simulink model "MotorAsincronoMotorCC1"  (Simulink 8.5)
settings: Solver=ode23t  StartTime=0.0  StopTime=3  RelTol=1e-3
undefined symbols (not defined in the file): powergui
libraries: powerlib x28, powerlib_extras x3
settings Model: Creator=RS  LastModifiedBy=Diego Cisternas
settings OptimizationCC: ExpressionDepthLimit=128  InitFltsAndDblsToZero=on
settings DebuggingCC: SaveWithParameterizedLinksMsg=none  SignalResolutionControl=TryResolveAllWithWarning  SolverPrmCheckMsg=warning  FcnCallInpInsideContextMsg=UseLocalSettings  StateNameClashWarn=none  StrictBusMsg=Warning
settings GRTTargetCC: TargetFcnLib=ansi_tfl_tmw.mat

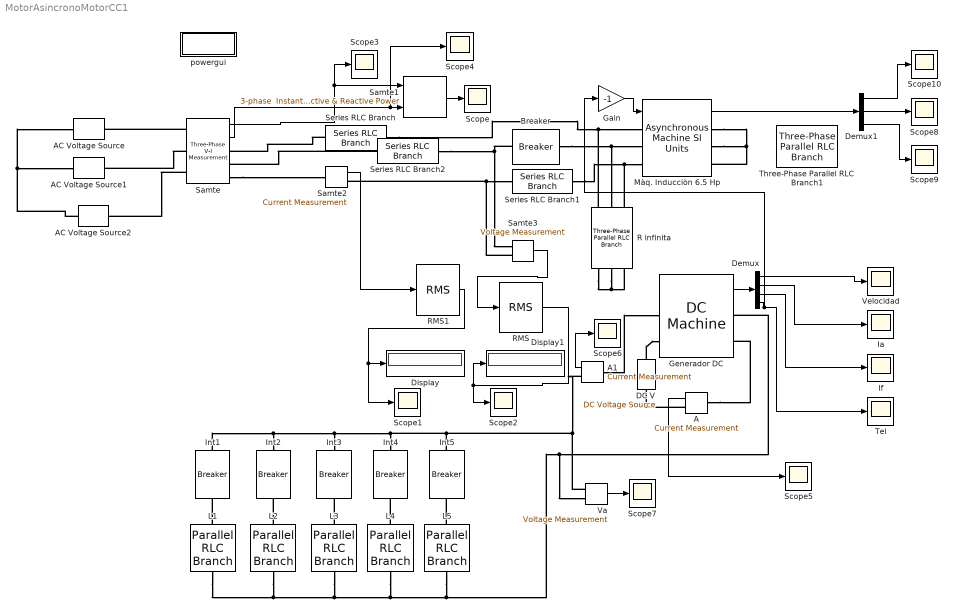
== system MotorAsincronoMotorCC1 ==
  A : powerlib/Measurements/Current Measurement  PhasorSimulation=off  OutputType=Complex  PSBequivalent=0
  A1 : powerlib/Measurements/Current Measurement  PhasorSimulation=off  OutputType=Complex  PSBequivalent=0
  AC Voltage Source : powerlib/Electrical Sources/AC Voltage Source  Amplitude=220.7*sqrt(2)  Phase=0  Frequency=50  SampleTime=0  Measurements=None
  AC Voltage Source1 : powerlib/Electrical Sources/AC Voltage Source  Amplitude=218.7*sqrt(2)  Phase=-119.5  Frequency=50  SampleTime=0  Measurements=None
  AC Voltage Source2 : powerlib/Electrical Sources/AC Voltage Source  Amplitude=220.7*sqrt(2)  Phase=121.3  Frequency=50  SampleTime=0  Measurements=None
  Breaker : powerlib/Elements/Breaker  InitialState=1  SwitchingTimes=0.7  External=off  BreakerResistance=0.01  SnubberResistance=1e6  SnubberCapacitance=inf  Measurements=None  MoreParameters=off  NoBreakLoop=off
  DC V : powerlib/Electrical Sources/DC Voltage Source  Amplitude=190  Measurements=None
  Demux : Demux
  Demux1 : Demux  Outputs=3
  Display : Display
  Display1 : Display
  Gain : Gain  Gain=-1
  Generador DC : powerlib/Machines/DC Machine  PresetModel=No  MechanicalLoad=Speed w  FieldType=Wound  ShowDetailedParameters=on  MeasurementBus=off  RLa="[ 0.5  0.01]"  RLf="[ 240  120]"  Laf=1.8  MachineConstant=Torque constant (N.m/A)  Ke=1.8  Kt=1.8  J=0.05  Bm=0.02  Tf=0  w0=0  Ifinit=1  TsPowergui=0  TsBlock=-1
  Ia : Scope
      settings: TimeRange=3  SaveName=ScopeData4  MaxDataPoints=10000000  SampleInput=on  SampleTime=10e-6
  If : Scope
      settings: SaveName=ScopeData5  MaxDataPoints=10000000  SampleInput=on  SampleTime=10e-6
  Int1 : powerlib/Elements/Breaker  InitialState=0  SwitchingTimes=0  External=off  BreakerResistance=0.01  SnubberResistance=1e6  SnubberCapacitance=inf  Measurements=None  MoreParameters=off  NoBreakLoop=off
  Int{2..5} (4 alike) : powerlib/Elements/Breaker  InitialState=0  SwitchingTimes=5  External=off  BreakerResistance=0.01  SnubberResistance=1e6  SnubberCapacitance=inf  Measurements=None  MoreParameters=off  NoBreakLoop=off
  L1 : powerlib/Elements/Parallel RLC Branch  LConnTagsString=a  RConnTagsString=__new0  BranchType=R  Resistance=20  Inductance=1e-3  SetiL0=off  InitialCurrent=0  Capacitance=1e-6  Setx0=off  InitialVoltage=0  Measurements=None
  L{2..5} (4 alike) : powerlib/Elements/Parallel RLC Branch  LConnTagsString=a  RConnTagsString=__new0  BranchType=R  Resistance=40  Inductance=1e-3  SetiL0=off  InitialCurrent=0  Capacitance=1e-6  Setx0=off  InitialVoltage=0  Measurements=None
  Màq. Inducciòn 6.5 Hp : powerlib/Machines/Asynchronous Machine SI Units  RotorType=Wound  PresetModel=No  MechanicalLoad=Torque Tm  ShowDetailedParameters=on  ReferenceFrame=Stationary  Units=SI  MeasurementBus=off  NominalParameters="[6.5*746    380   50]"  Stator="[0.03   0.00006]"  Rotor="[1.094  0.00496]"  Cage1=[0.4155 0.002066]  Cage2=[0.4168 0.0003495]  Lm=0.105  Mechanical="[0.041    0.001   2]"  PolePairs=2  InitialConditions="[ 1,0   0,0,0   0,0,0 ]"  SimulateSaturation=on  Saturation=[ 0.5 3,6,9,12,15,18,30,50;20,190,380,400,420,440,450,451,452]  LoadFlowParameters=0  TsPowergui=0  TsBlock=-1  IterativeModel=Trapezoidal non iterative  Pmec=1.492e+006
  R infinita : powerlib/Elements/Three-Phase Parallel RLC Branch  LConnTagsString=A|B|C  RConnTagsString=A|B|C  BranchType=R  Resistance=1000000  Inductance=1e-3  Capacitance=1e-6  Measurements=None
  RMS : powerlib_extras/Measurements/RMS  f1=50
  RMS1 : powerlib_extras/Measurements/RMS  f1=50
  Samte : powerlib/Measurements/Three-Phase V-I Measurement  VoltageMeasurement=phase-to-phase  SetLabelV=off  LabelV=Vabc  Vpu=off  VpuLL=off  CurrentMeasurement=yes  SetLabelI=off  LabelI=Iabc  Ipu=off  Pbase=100e6  Vbase=500e3  OutputType=Complex  PhasorSimulation=off  PSBequivalent=0
  Samte1 : powerlib_extras/Measurements/3-phase  Instantaneous  Active & Reactive Power
  Samte2 : powerlib/Measurements/Current Measurement  PhasorSimulation=off  OutputType=Complex  PSBequivalent=0
  Samte3 : powerlib/Measurements/Voltage Measurement  PhasorSimulation=off  OutputType=Complex  PSBequivalent=0
  Scope{,1..10} (11 alike) : Scope
      Scope settings: MaxDataPoints=10000000  SampleInput=on  SampleTime=10e-6
      Scope1 settings: MaxDataPoints=10000000  SampleInput=on  SampleTime=10e-6
      Scope10 settings: SaveName=ScopeData14  MaxDataPoints=10000000  SampleInput=on  SampleTime=10e-6
      Scope2 settings: YMin=378.99  YMax=378.99  SaveName=ScopeData2  MaxDataPoints=10000000  SampleInput=on  SampleTime=10e-6
      Scope3 settings: SaveName=ScopeData10  MaxDataPoints=10000000  SampleInput=on  SampleTime=10e-6
      Scope4 settings: TimeRange=3  SaveName=ScopeData11  MaxDataPoints=10000000  SampleInput=on  SampleTime=10e-6
      Scope5 settings: YMin=-0.791667  YMax=-0.791667  SaveName=ScopeData12  MaxDataPoints=10000000  SampleInput=on  SampleTime=10e-6
      Scope6 settings: YMin=10.588  YMax=10.598  SaveName=ScopeData13  MaxDataPoints=10000000  SampleInput=on  SampleTime=10e-6
      Scope7 settings: YMin=168.4  YMax=169.9  SaveName=ScopeData7  MaxDataPoints=10000000  SampleInput=on  SampleTime=10e-6
      Scope8 settings: SaveName=ScopeData8  MaxDataPoints=10000000  SampleInput=on  SampleTime=10e-6
      Scope9 settings: SaveName=ScopeData9  MaxDataPoints=10000000  SampleInput=on  SampleTime=10e-6
  Series RLC Branch : powerlib/Elements/Series RLC Branch  LConnTagsString=__new0  RConnTagsString=__new0  BranchType=RL  Resistance=0.6  Inductance=0.0049  SetiL0=off  InitialCurrent=0  Capacitance=1e-6  Setx0=off  InitialVoltage=0  Measurements=None
  Series RLC Branch1 : powerlib/Elements/Series RLC Branch  LConnTagsString=__new0  RConnTagsString=__new0  BranchType=RL  Resistance=0.6  Inductance=0.0049  SetiL0=off  InitialCurrent=0  Capacitance=1e-6  Setx0=off  InitialVoltage=0  Measurements=None
  Series RLC Branch2 : powerlib/Elements/Series RLC Branch  LConnTagsString=__new0  RConnTagsString=__new0  BranchType=RL  Resistance=0.6  Inductance=0.0049  SetiL0=off  InitialCurrent=0  Capacitance=1e-6  Setx0=off  InitialVoltage=0  Measurements=None
  Tel : Scope
      settings: SaveName=ScopeData6  MaxDataPoints=10000000  SampleInput=on  SampleTime=10e-6
  Three-Phase Parallel RLC Branch1 : powerlib/Elements/Three-Phase Parallel RLC Branch  LConnTagsString=A|B|C  RConnTagsString=A|B|C  BranchType=R  Resistance=4.2  Inductance=1e-3  Capacitance=1e-6  Measurements=None
  Va : powerlib/Measurements/Voltage Measurement  PhasorSimulation=off  OutputType=Complex  PSBequivalent=0
  Velocidad : Scope
      settings: SaveName=ScopeData3  MaxDataPoints=10000000  SampleInput=on  SampleTime=10e-6
  powergui : Subsystem  AncestorBlock=powerlib/powergui  InitFcn=powergui( 'InitFcn_Callback' , gcb , 0 , [ ] );  mask(PSB option menu block){SimulationMode=Continuous, SampleTime=50e-6, echomessages=off, RestoreLinks=warning, x0status=blocks, Frange=[0:2:500], Ylog=off, Xlog=on, ShowGrid=off, save=off, variable=ZData, structure=, ZoomFFT=on, StartTime=0.0, cycles=1, DisplayStyle=1, fundamental=60, FreqAxis=off, MaxFrequency=1000, frequencyindice=50, frequencyindicesteady=1, RmsSteady=1, display=off, Ts=0, frequency=60, methode=off, HookPort=off, Interpol=off}
      mask prompts: SimulationMode "Simulation mode"; SampleTime "Sample time Ts (when simulation mode is Discrete) (s)"; echomessages "Echo  Messages"; RestoreLinks "Restore disabled links"; x0status "Initial electrical states status"; Frange "Impedance tool: Frequency Range"; Ylog "Impedance tool: Log impedance"; Xlog "Impedance tool: log Frequency"; ShowGrid "Impedance tool: grid"; save "Impedance tool: Save Data To Workspace"; variable "Impedance tool: Variable Name"; structure "Structure Name (PSBFFTSCOPE)"; ZoomFFT "ZoomFFT (PSBFFTSCOPE)"; StartTime "Start Time (PSBFFTSCOPE)"; cycles "Cycles (PSBFFTSCOPE)"; DisplayStyle "Display style (PSBFFTSCOPE)"; fundamental "Fundamental (PSBFFTSCOPE)"; FreqAxis "Frequency Axis (PSBFFTSCOPE)"; MaxFrequency "Max Frequency (PSBFFTSCOPE)"; frequencyindice "Load flow frequency (Hz)"; frequencyindicesteady "Frequency indice (STEADYSTATE)"; RmsSteady "RMS display (STEADYSTATE)"; display "Display Results"; Ts "OBSOLETE 1"; frequency "Phasor frequency (Hz)"; methode "Phasor simulation"; HookPort "Hook port"; Interpol "Interpolate"
      mask init:
      | powerlibroot = which('powersysdomain');
      | PSBroot = powerlibroot(1:end-16);
      | %
      | switch SimulationMode
      | 	case 1
      | 		message=sprintf('Continuous');
      | 	case 2
      |         SampleTimeeval=evalin('base',SampleTime,'NaN');
      |         if isnan(SampleTimeeval)
      |             message=sprintf('Warning !!,\nUndefined sample time');
      |         else
      |             message=sprintf('Discrete,\nTs = %.4g s.',SampleTimeeval);
      |         end
      | 	case 3
      | 		message=sprintf('Phasors');
      | end
      | if strcmp(bdroot,'powerlib')
      |   message='powergui';
      | end
      | power_initmask();
      settings: CopyFcn=powergui( 'Copy_Callback' , gcb , 0 , [ ] );  ModelCloseFcn=powergui( 'CloseButton_Callback' , gcb , [ ] , [ ] );  PreSaveFcn=powergui( 'CloseButton_Callback' , gcb , [ ] , [ ] );  NameChangeFcn=powergui( 'NameChangeFcn_Callback' , gcb , 0 , [ ] );
      settings: DeleteFcn=|
      | powergui( 'Copy_Callback' , gcb , 1 , [ ] );
      | powergui( 'CloseButton_Callback' , gcb , [ ] , [ ] );
      settings: OpenFcn=|
      | if (power_openblockproxy ('secondary'))
      | powergui(gcb,'PM')
      | end;
      mask Help: web(psbhelp)
      mask TypeOptions SimulationMode: Continuous | Discrete | Phasor
      mask TypeOptions RestoreLinks: yes | warning | no
      mask TypeOptions x0status: blocks | steady | zero
      mask Callback HookPort: powergui('HookPort',[],[],gcb);
      mask Display: disp(message)
  wires:
  Samte/1 -> Samte1/1, Scope3/1
  Samte/2 -> Samte1/2, Scope4/1
  Samte3/1 -> RMS/1
  RMS/1 -> Display1/1, Scope2/1
  Samte1/1 -> Scope/1
  Màq. Inducciòn 6.5 Hp/1 -> Demux1/1
  Generador DC/1 -> Demux/1
  Gain/1 -> Màq. Inducciòn 6.5 Hp/1
  Demux/4 -> Tel/1, Gain/1
  Demux/1 -> Velocidad/1
  Demux/2 -> Ia/1
  Demux/3 -> If/1
  Va/1 -> Scope7/1
  RMS1/1 -> Display/1, Scope1/1
  A/1 -> Scope5/1
  A1/1 -> Scope6/1
  Demux1/1 -> Scope10/1
  Samte2/1 -> RMS1/1
  Demux1/2 -> Scope8/1
  Demux1/3 -> Scope9/1
  connections:
  Breaker/LConn1 -- Series RLC Branch2/RConn1 -- Samte3/LConn1
  R infinita/LConn1 -- Series RLC Branch/RConn1 -- Màq. Inducciòn 6.5 Hp/LConn1
  Samte/LConn3 -- AC Voltage Source2/RConn1
  Samte/RConn3 -- Samte2/LConn1
  R infinita/LConn3 -- Màq. Inducciòn 6.5 Hp/LConn3 -- Series RLC Branch1/RConn1
  DC V/RConn1 -- Generador DC/LConn2
  L1/LConn1 -- Int1/RConn1
  L2/LConn1 -- Int2/RConn1
  L3/LConn1 -- Int3/RConn1
  L4/LConn1 -- Int4/RConn1
  L5/LConn1 -- Int5/RConn1
  L1/RConn1 -- L2/RConn1 -- L3/RConn1 -- L4/RConn1 -- L5/RConn1 -- Generador DC/RConn1 -- Va/LConn2
  Va/LConn1 -- A1/RConn1 -- Int1/LConn1 -- Int2/LConn1 -- Int3/LConn1 -- Int4/LConn1 -- Int5/LConn1
  R infinita/RConn1 -- R infinita/RConn3 -- R infinita/RConn2
  A/RConn1 -- DC V/LConn1
  A/LConn1 -- Generador DC/RConn2
  AC Voltage Source2/LConn1 -- AC Voltage Source/LConn1 -- AC Voltage Source1/LConn1
  Samte/LConn1 -- AC Voltage Source/RConn1
  Samte/LConn2 -- AC Voltage Source1/RConn1
  A1/LConn1 -- Generador DC/LConn1
  Breaker/RConn1 -- Màq. Inducciòn 6.5 Hp/LConn2 -- R infinita/LConn2
  Màq. Inducciòn 6.5 Hp/RConn1 -- Màq. Inducciòn 6.5 Hp/RConn3 -- Màq. Inducciòn 6.5 Hp/RConn2
  Series RLC Branch/LConn1 -- Samte/RConn1
  Samte3/LConn2 -- Series RLC Branch1/LConn1 -- Samte2/RConn1
  Series RLC Branch2/LConn1 -- Samte/RConn2

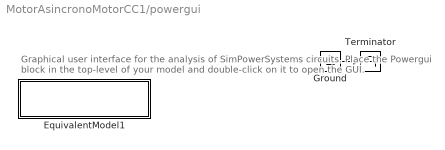
== system MotorAsincronoMotorCC1/powergui ==
  note: Graphical user interface for the analysis of  SimPowerSystems circuits.
      | Place the Powergui block in the top-level of your model and double-click
      | on it to open the GUI.
  EquivalentModel1 : Subsystem
      mask init:
      | SPS = get_param(gcbh,'UserData');
      | if isempty(SPS)
      |     A=0;
      |     B=0;
      |     C=0;
      |     D=0;
      |     x0=0;
      |     SwitchResistance=1;
      |     SwitchType=1;
      |     SwitchGateInitialValue=1;
      |     OutputsToResetToZero=1;
      | else
      | 	A=SPS.A;
      |     B=SPS.B;
      |     C=SPS.C;
      |     D=SPS.D;
      |     x0=SPS.x0;
      |     SwitchResistance=SPS.SwitchResistance;
      |     SwitchType=SPS.SwitchType;
      |     SwitchGateInitialValue=SPS.SwitchGateInitialValue;
      |     OutputsToResetToZero=SPS.YSwitchCurrent;
      | end
      mask Display:
      | color('blue')
      | disp('EQUIVALENT CIRCUIT')
  Ground : Ground
  Terminator : Terminator
  wires:
  Ground/1 -> Terminator/1

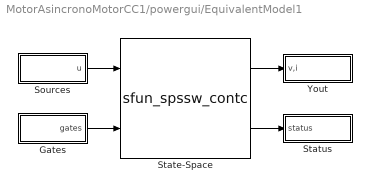
== system MotorAsincronoMotorCC1/powergui/EquivalentModel1 ==
  Gates : Subsystem
  Sources : Subsystem
  State-Space : S-Function  FunctionName=sfun_spssw_contc  Parameters=A, B, C, D, x0, SwitchResistance ,SwitchType, SwitchGateInitialValue, OutputsToResetToZero
  Status : Subsystem
  Yout : Subsystem
  wires:
  Gates/1(gates) -> State-Space/2
  Sources/1(u) -> State-Space/1
  State-Space/2 -> Status/1(status)
  State-Space/1 -> Yout/1(v,i)

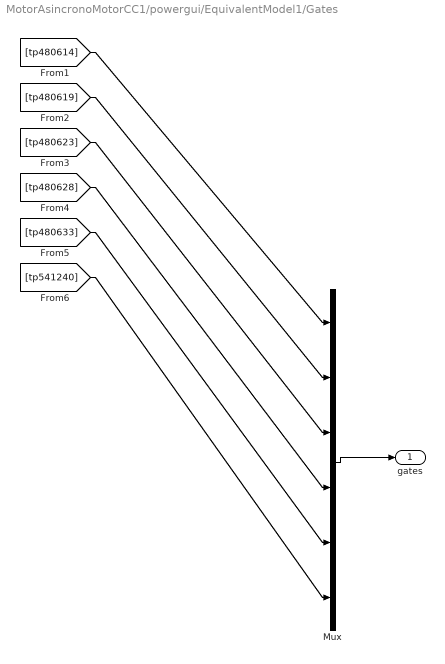
== system MotorAsincronoMotorCC1/powergui/EquivalentModel1/Gates ==
  Mux : Mux  Inputs=[1 1 1 1 1 1]
  gates : Outport
  wires:
  Mux/1 -> gates/1
  [tp480614] -> Mux/1
  [tp480619] -> Mux/2
  [tp480623] -> Mux/3
  [tp480628] -> Mux/4
  [tp480633] -> Mux/5
  [tp541240] -> Mux/6

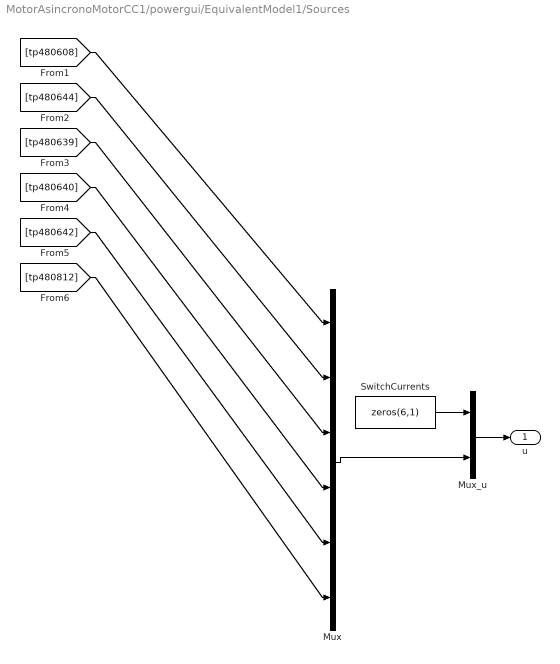
== system MotorAsincronoMotorCC1/powergui/EquivalentModel1/Sources ==
  Mux : Mux  Inputs=[4 1 1 1 1 1]
  Mux_u : Mux  Inputs=[6 9]
  SwitchCurrents : Constant  Value=zeros(6,1)
  u : Outport
  wires:
  Mux/1 -> Mux_u/2
  SwitchCurrents/1 -> Mux_u/1
  Mux_u/1 -> u/1
  [tp480608] -> Mux/1
  [tp480644] -> Mux/2
  [tp480639] -> Mux/3
  [tp480640] -> Mux/4
  [tp480642] -> Mux/5
  [tp480812] -> Mux/6

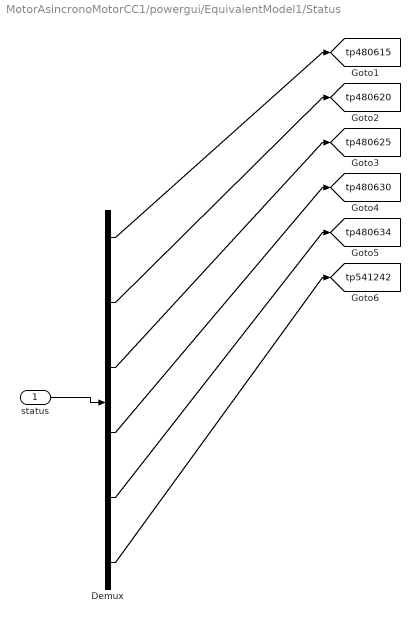
== system MotorAsincronoMotorCC1/powergui/EquivalentModel1/Status ==
  status : Inport
  Demux : Demux  Outputs=[1 1 1 1 1 1]
  tag scope: tp480615=global, tp480620=global, tp480625=global, tp480630=global, tp480634=global, tp541242=global
  wires:
  status/1 -> Demux/1
  Demux/1 -> [tp480615]
  Demux/2 -> [tp480620]
  Demux/3 -> [tp480625]
  Demux/4 -> [tp480630]
  Demux/5 -> [tp480634]
  Demux/6 -> [tp541242]

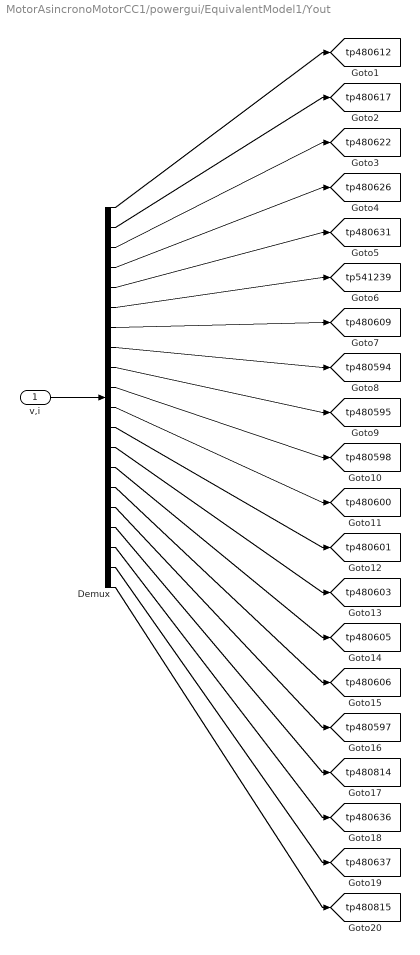
== system MotorAsincronoMotorCC1/powergui/EquivalentModel1/Yout ==
  v,i : Inport
  Demux : Demux  Outputs=[1 1 1 1 1 1 4 1 1 1 1 1 1 1 1 1 1 1 1 1]
  tag scope: tp480594=global, tp480595=global, tp480597=global, tp480598=global, tp480600=global, tp480601=global, tp480603=global, tp480605=global, tp480606=global, tp480609=global, tp480612=global, tp480617=global, tp480622=global, tp480626=global, tp480631=global, tp480636=global, tp480637=global, tp480814=global, tp480815=global, tp541239=global
  wires:
  v,i/1 -> Demux/1
  Demux/1 -> [tp480612]
  Demux/2 -> [tp480617]
  Demux/3 -> [tp480622]
  Demux/4 -> [tp480626]
  Demux/5 -> [tp480631]
  Demux/6 -> [tp541239]
  Demux/7 -> [tp480609]
  Demux/8 -> [tp480594]
  Demux/9 -> [tp480595]
  Demux/10 -> [tp480598]
  Demux/11 -> [tp480600]
  Demux/12 -> [tp480601]
  Demux/13 -> [tp480603]
  Demux/14 -> [tp480605]
  Demux/15 -> [tp480606]
  Demux/16 -> [tp480597]
  Demux/17 -> [tp480814]
  Demux/18 -> [tp480636]
  Demux/19 -> [tp480637]
  Demux/20 -> [tp480815]
